simulink model "Soal1"  (R2021b)
settings: Solver=VariableStepAuto  StartTime=0.0  StopTime=10.0  RelTol=1e-3
settings Model: Creator=Parsa  LastModifiedBy=Parsa

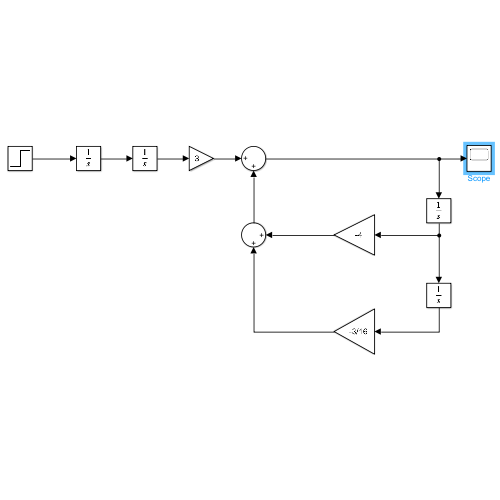
[thumbnail: Simulink's stored preview of the top-level diagram]
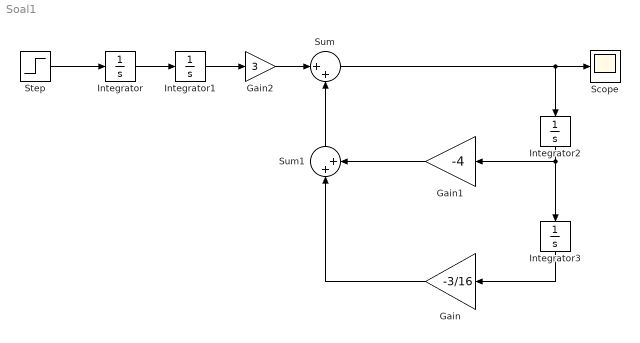
== system Soal1 ==
  Gain : Gain  Gain=-3/16
  Gain1 : Gain  Gain=-4
  Gain2 : Gain  Gain=3
  Integrator{,1..3} (4 alike) : Integrator
  Scope : Scope
  Step : Step  Time=0.001  SampleTime=0
  Sum : Sum  Inputs=|++
  Sum1 : Sum  Inputs=|++
  wires:
  Integrator/1 -> Integrator1/1
  Step/1 -> Integrator/1
  Integrator1/1 -> Gain2/1
  Sum/1 -> Integrator2/1, Scope/1
  Integrator2/1 -> Integrator3/1, Gain1/1
  Integrator3/1 -> Gain/1
  Gain1/1 -> Sum1/2
  Sum1/1 -> Sum/2
  Gain/1 -> Sum1/1
  Gain2/1 -> Sum/1
